simulink subsystem "energyBalance"  (R2024a)
settings: Solver=VariableStepAuto  StartTime=0.0  StopTime=2568180  RelTol=1e-3
settings Model: DefaultTestHarness=energyBalance_HarnessFromWorkspace  Creator=eunice.duplessis  LastModifiedBy=jason.miskin

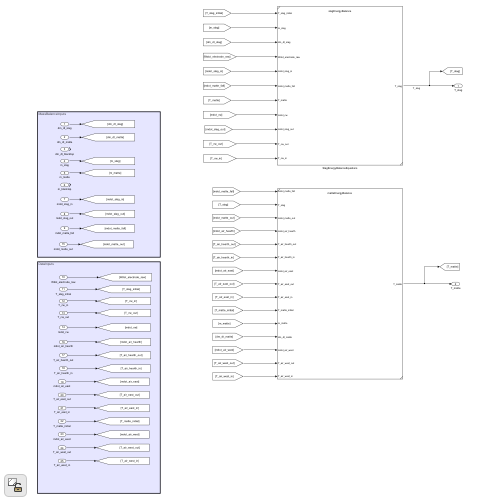
[thumbnail: Simulink's stored preview of the top-level diagram]
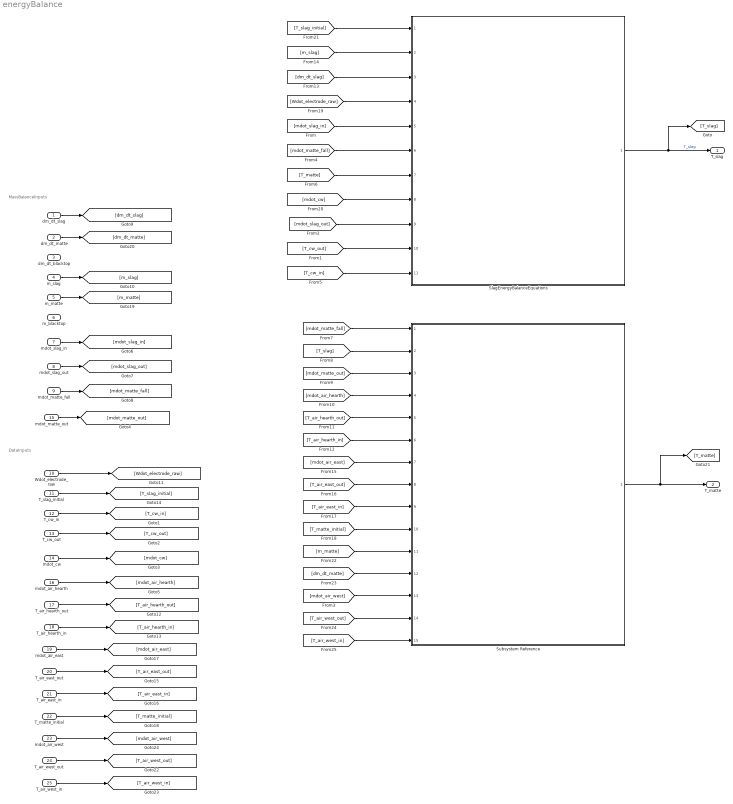
== system energyBalance ==
  note: MassBalanceInputs
  note: DataInputs
  dm_dt_slag : Inport
  dm_dt_matte : Inport  Port=2
  dm_dt_blacktop : Inport  Port=3
  m_slag : Inport  Port=4
  m_matte : Inport  Port=5
  m_blacktop : Inport  Port=6
  mdot_slag_in : Inport  Port=7
  mdot_slag_out : Inport  Port=8
  mdot_matte_fall : Inport  Port=9
  Wdot_electrode_raw : Inport  Port=10
  T_slag_initial : Inport  Port=11
  T_cw_in : Inport  Port=12
  T_cw_out : Inport  Port=13
  mdot_cw : Inport  Port=14
  mdot_matte_out : Inport  Port=15
  mdot_air_hearth : Inport  Port=16
  T_air_hearth_out : Inport  Port=17
  T_air_hearth_in : Inport  Port=18
  mdot_air_east : Inport  Port=19
  T_air_east_out : Inport  Port=20
  T_air_east_in : Inport  Port=21
  T_matte_initial : Inport  Port=22
  mdot_air_west : Inport  Port=23
  T_air_west_out : Inport  Port=24
  T_air_west_in : Inport  Port=25
  SlagEnergyBalanceEquations : Subsystem  ReferencedSubsystem=slagEnergyBalance
      settings: PermitHierarchicalResolution=None
  Subsystem Reference : Subsystem  ReferencedSubsystem=matteEnergyBalance
      settings: PermitHierarchicalResolution=None
  T_slag : Outport
  T_matte : Outport  Port=2
  wires:
  mdot_slag_in/1 -> [mdot_slag_in]
  mdot_slag_out/1 -> [mdot_slag_out]
  mdot_matte_fall/1 -> [mdot_matte_fall]
  dm_dt_slag/1 -> [dm_dt_slag]
  m_slag/1 -> [m_slag]
  Wdot_electrode_raw/1 -> [Wdot_electrode_raw]
  T_slag_initial/1 -> [T_slag_initial]
  [T_slag_initial] -> SlagEnergyBalanceEquations/1
  [m_slag] -> SlagEnergyBalanceEquations/2
  [dm_dt_slag] -> SlagEnergyBalanceEquations/3
  [Wdot_electrode_raw] -> SlagEnergyBalanceEquations/4
  [mdot_slag_in] -> SlagEnergyBalanceEquations/5
  [mdot_matte_fall] -> SlagEnergyBalanceEquations/6
  [T_matte] -> SlagEnergyBalanceEquations/7
  [mdot_cw] -> SlagEnergyBalanceEquations/8
  [mdot_slag_out] -> SlagEnergyBalanceEquations/9
  SlagEnergyBalanceEquations/1 -> T_slag/1, [T_slag]  "T_slag"
  T_cw_in/1 -> [T_cw_in]
  T_cw_out/1 -> [T_cw_out]
  mdot_cw/1 -> [mdot_cw]
  [T_cw_out] -> SlagEnergyBalanceEquations/10
  [T_cw_in] -> SlagEnergyBalanceEquations/11
  [mdot_matte_fall] -> Subsystem Reference/1
  [T_slag] -> Subsystem Reference/2
  mdot_matte_out/1 -> [mdot_matte_out]
  [mdot_matte_out] -> Subsystem Reference/3
  mdot_air_hearth/1 -> [mdot_air_hearth]
  [mdot_air_hearth] -> Subsystem Reference/4
  T_air_hearth_out/1 -> [T_air_hearth_out]
  [T_air_hearth_out] -> Subsystem Reference/5
  T_air_hearth_in/1 -> [T_air_hearth_in]
  [T_air_hearth_in] -> Subsystem Reference/6
  T_air_east_in/1 -> [T_air_east_in]
  T_air_east_out/1 -> [T_air_east_out]
  mdot_air_east/1 -> [mdot_air_east]
  [mdot_air_east] -> Subsystem Reference/7
  [T_air_east_out] -> Subsystem Reference/8
  [T_air_east_in] -> Subsystem Reference/9
  T_matte_initial/1 -> [T_matte_initial]
  [T_matte_initial] -> Subsystem Reference/10
  m_matte/1 -> [m_matte]
  [m_matte] -> Subsystem Reference/11
  [dm_dt_matte] -> Subsystem Reference/12
  dm_dt_matte/1 -> [dm_dt_matte]
  Subsystem Reference/1 -> T_matte/1, [T_matte]
  mdot_air_west/1 -> [mdot_air_west]
  T_air_west_out/1 -> [T_air_west_out]
  T_air_west_in/1 -> [T_air_west_in]
  [T_air_west_out] -> Subsystem Reference/14
  [mdot_air_west] -> Subsystem Reference/13
  [T_air_west_in] -> Subsystem Reference/15
